simulink library "otk"  (Simulink 8.1)
settings: Solver=ode45  StartTime=0.0  StopTime=10.0  RelTol=1e-3
undefined symbols (not defined in the file or in its folder): C_TICK_TIME_S, FALSE, KIFO_DriverOvertakeTimer_ms, KIFO_MinOvertakeSpd_kph, KIFO_MinRelOvertakeSpd_kph, TRUE, ZERO_INT
libraries: tsl x1, tsr x1, hcu_lib x1
settings Model: Creator=xsellart  LastModifiedBy=AT015555

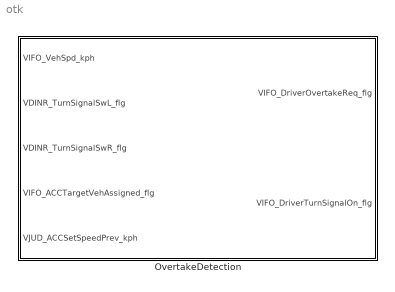
== system otk ==
  OvertakeDetection : Subsystem

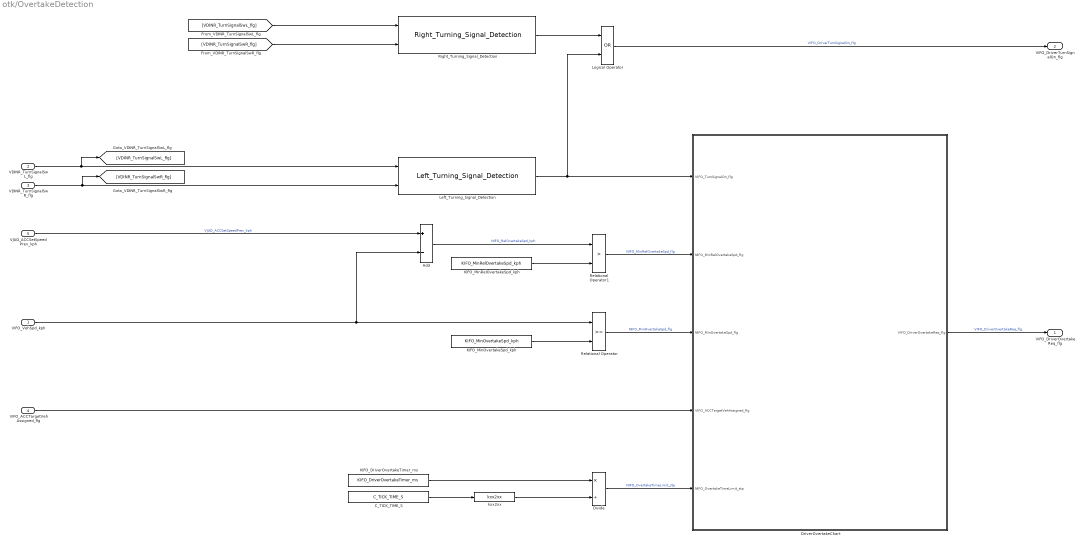
== system otk/OvertakeDetection ==
  VIFO_VehSpd_kph : Inport
  VDINR_TurnSignalSwL_flg : Inport  Port=2
  VDINR_TurnSignalSwR_flg : Inport  Port=3
  VIFO_ACCTargetVehAssigned_flg : Inport  Port=4
  VJUD_ACCSetSpeedPrev_kph : Inport  Port=5
  Add : Sum  Inputs=+-  OutDataTypeStr=Inherit: Inherit via back propagation
  C_TICK_TIME_S : Constant  Value=C_TICK_TIME_S  OutDataTypeStr=single
  Divide : Product  Inputs=*/
  DriverOvertakeChart : Stateflow chart  TreatAsAtomicUnit=on
  KIFO_DriverOvertakeTimer_ms : Constant  Value=KIFO_DriverOvertakeTimer_ms  OutDataTypeStr=single
  KIFO_MinOvertakeSpd_kph : Constant  Value=KIFO_MinOvertakeSpd_kph  OutDataTypeStr=single
  KIFO_MinRelOvertakeSpd_kph : Constant  Value=KIFO_MinRelOvertakeSpd_kph  OutDataTypeStr=single
  Left_Turning_Signal_Detection : tsl/Left_Turning_Signal_Detection
  Logical Operator : Logic  Operator=OR  AllPortsSameDT=off  OutDataTypeStr=boolean
  Relational Operator : RelationalOperator  OutDataTypeStr=boolean
  Relational Operator1 : RelationalOperator  Operator=>  OutDataTypeStr=boolean
  Right_Turning_Signal_Detection : tsr/Right_Turning_Signal_Detection
  kxx2xx : hcu_lib/kxx2xx
  VIFO_DriverOvertakeReq_flg : Outport
  VIFO_DriverTurnSignalOn_flg : Outport  Port=2
  wires:
  VDINR_TurnSignalSwR_flg/1 -> [VDINR_TurnSignalSwR_flg], Left_Turning_Signal_Detection/2
  Left_Turning_Signal_Detection/1 -> Logical Operator/2, DriverOvertakeChart/1(VIFO_TurnSignalOn_flg)
  VDINR_TurnSignalSwL_flg/1 -> [VDINR_TurnSignalSwL_flg], Left_Turning_Signal_Detection/1
  VJUD_ACCSetSpeedPrev_kph/1 -> Add/1  "VJUD_ACCSetSpeedPrev_kph"
  KIFO_MinRelOvertakeSpd_kph/1 -> Relational Operator1/2
  Relational Operator1/1 -> DriverOvertakeChart/2(NIFO_MinRelOvertakeSpd_flg)  "NIFO_MinRelOvertakeSpd_flg"
  Add/1 -> Relational Operator1/1  "NIFO_RelOvertakeSpd_kph"
  VIFO_ACCTargetVehAssigned_flg/1 -> DriverOvertakeChart/4(VIFO_ACCTargetVehAssigned_flg)
  Relational Operator/1 -> DriverOvertakeChart/3(NIFO_MinOvertakeSpd_flg)  "NIFO_MinOvertakeSpd_flg"
  KIFO_MinOvertakeSpd_kph/1 -> Relational Operator/2
  VIFO_VehSpd_kph/1 -> Add/2, Relational Operator/1
  kxx2xx/1 -> Divide/2
  Divide/1 -> DriverOvertakeChart/5(NIFO_OvertakeTimeLimit_stp)  "NIFO_OvertakeTimeLimit_stp"
  C_TICK_TIME_S/1 -> kxx2xx/1
  KIFO_DriverOvertakeTimer_ms/1 -> Divide/1
  DriverOvertakeChart/1(VIFO_DriverOvertakeReq_flg) -> VIFO_DriverOvertakeReq_flg/1  "VIFO_DriverOvertakeReq_flg"
  [VDINR_TurnSignalSwL_flg] -> Right_Turning_Signal_Detection/1
  [VDINR_TurnSignalSwR_flg] -> Right_Turning_Signal_Detection/2
  Right_Turning_Signal_Detection/1 -> Logical Operator/1
  Logical Operator/1 -> VIFO_DriverTurnSignalOn_flg/1  "VIFO_DriverTurnSignalOn_flg"

== stateflow chart OvertakeDetection/DriverOvertakeChart ==
  state OFF
    en:
    VIFO_DriverOvertakeReq_flg = FALSE;
  state OVERTAKE
    en:
    VIFO_DriverOvertakeReq_flg = TRUE;
    NIFO_OvertakeTimeLocal_stp = ZERO_INT;
    du:
    NIFO_OvertakeTimeLocal_stp=NIFO_OvertakeTimeLocal_stp+1;
  state OVERTAKE_OVERFLOW
    en:
    VIFO_DriverOvertakeReq_flg = FALSE;
  (default) -> state3
  state3 -> OVERTAKE : [VIFO_TurnSignalOn_flg==TRUE...
      | && NIFO_MinOvertakeSpd_flg==TRUE...
      | && NIFO_MinRelOvertakeSpd_flg==TRUE...
      | && VIFO_ACCTargetVehAssigned_flg == TRUE]
  OVERTAKE -> OVERTAKE_OVERFLOW [order 2] : [ NIFO_OvertakeTimeLocal_stp >= NIFO_OvertakeTimeLimit_stp]
  OVERTAKE -> state3 [order 1] : [ VIFO_TurnSignalOn_flg == FALSE ...
      | || VIFO_ACCTargetVehAssigned_flg == FALSE]
  OVERTAKE_OVERFLOW -> (junction 16)
  (junction 16) -> state3 : [ VIFO_TurnSignalOn_flg == FALSE ...
      | || VIFO_ACCTargetVehAssigned_flg == FALSE]
  data: VIFO_DriverOvertakeReq_flg output boolean; VIFO_TurnSignalOn_flg input boolean; NIFO_MinRelOvertakeSpd_flg input double; NIFO_MinOvertakeSpd_flg input boolean; FALSE parameter double; TRUE parameter double; VIFO_ACCTargetVehAssigned_flg input double; NIFO_OvertakeTimeLocal_stp local single; NIFO_OvertakeTimeLimit_stp input single; ZERO_INT parameter uint8
